simulink library "cpg_lib"  (R2016b)
settings: Solver=VariableStepAuto  StartTime=0.0  StopTime=10.0  RelTol=1e-3  EnableMultiTasking=on
undefined symbols (not defined in the file or in its folder): AFOFS_DIM, c, c_jointstop, CPG, D1G_HAT, DeltaThRef, eref, FmaxGAS, FmaxGLU, FmaxHAM, FmaxHFL, FmaxSOL, FmaxTA, FmaxVAS, GainDeltaTheta, GainGAS, GainGLU, GainHAM, GainHAMHFL, GainHFL, GainKneOverExt, GainSOL, GainSOLTA, GainTA, GainVAS, GroundFunction, K, K_swing, KneePh23Offset, LceOffsetHAM, LceOffsetHFL, LceOffsetTA, left, LongDelay, loptGAS, loptGLU, loptHAM, loptHFL, loptSOL, loptTA, loptVAS, lslackGAS, lslackGLU, lslackHAM, lslackHFL, lslackSOL, lslackTA, lslackVAS, massGAS, massGLU, massHAM, massHFL, massSOL, massTA, massVAS, MidDelay, N, N_record, N_start, phi12_LowLimit ... (+67)
undefined symbols (not defined in the file): NominalShape1
libraries: cpg_lib x36, simulink_extras x14, simulink x5, nmc x3
(part 1 of 4)
settings Model: Creator=efx  LastModifiedBy=brugtjh
settings DataIOCC: LimitDataPoints=on
settings OptimizationCC: LifeSpan=inf
settings DebuggingCC: AllowSymbolicDim=off  SFUnexpectedBacktrackingDiag=warning  SFNoUnconditionalDefaultTransitionDiag=warning  SFExecutionAtInitializationDiag=none
settings ModelReferenceCC: PropagateSignalLabelsOutOfModel=off
settings GRTTargetCC: TargetLangStandard=C89/C90 (ANSI)
settings ConfigComp: CovMetricSettings=dw  CovHtmlReporting=on  CovSaveCumulativeToWorkspaceVar=on  CovSaveSingleToWorkspaceVar=on  CovExternalEMLEnable=off

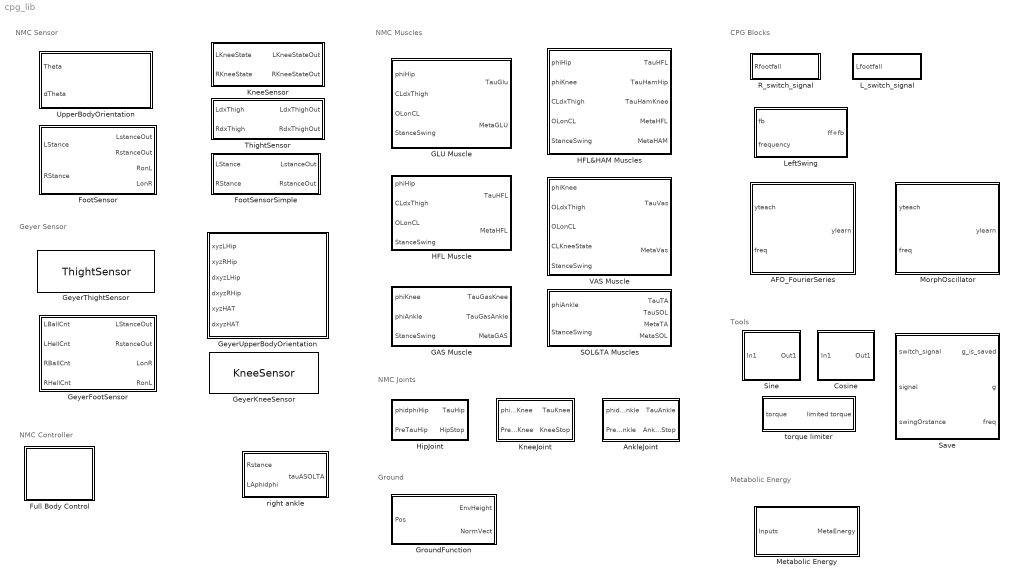
== system cpg_lib ==
  note: NMC Joints
  note: NMC Muscles
  note: Geyer Sensor
  note: NMC Sensor
  note: Tools
  note: CPG Blocks
  note: NMC Controller
  note: Metabolic Energy
  note: Ground
  AFO_FourierSeries : Subsystem
  AnkleJoint : Subsystem
  Cosine : Subsystem
  FootSensor : Subsystem
  FootSensorSimple : Subsystem
  Full Body Control : Subsystem
  GAS Muscle : Subsystem
  GLU Muscle : Subsystem
  GeyerFootSensor : Subsystem
  GeyerKneeSensor : cpg_lib/KneeSensor
  GeyerThightSensor : cpg_lib/ThightSensor
  GeyerUpperBodyOrientation : Subsystem
  GroundFunction : Subsystem
  "HFL Muscle " : Subsystem
  HFL&HAM Muscles : Subsystem
  HipJoint : Subsystem
  KneeJoint : Subsystem
  KneeSensor : Subsystem
  L_switch_signal : Subsystem
  LeftSwing : Subsystem  InitFcn=CPG.initCurrent();  StopFcn=CPG.saveCurrent();  mask{SaveName=NominalShape1}
      mask prompts: SaveName "Signal nominal shape name"
      mask init:
      | evalin('base','CPG.initCPG();');
      settings: CopyFcn=CPG.initCPG_automaticName();
  Metabolic Energy : Subsystem
  MorphOscillator : Subsystem
  R_switch_signal : Subsystem
  SOL&TA Muscles : Subsystem
  Save : Subsystem
  Sine : Subsystem
  ThightSensor : Subsystem
  UpperBodyOrientation : Subsystem
  VAS Muscle : Subsystem
  right ankle : Subsystem
  torque limiter : Subsystem

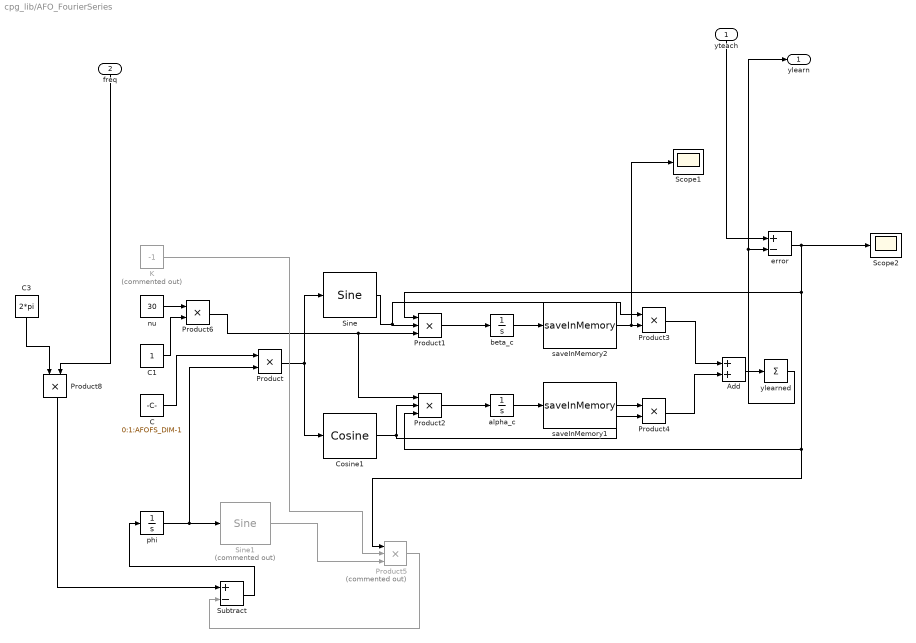
== system cpg_lib/AFO_FourierSeries ==
  yteach : Inport
  freq : Inport  Port=2
  Add : Sum
  C : Constant  Value=0:1:AFOFS_DIM-1
  C1 : Constant
  C3 : Constant  Value=2*pi
  Cosine1 : cpg_lib/Cosine
  K : Constant  Commented=on  Value=-1
  Product{,3..4,6,8} (5 alike) : Product
  Product1 : Product  Inputs=3
  Product2 : Product  Inputs=3
  Product5 : Product  Commented=on  Inputs=3
  Scope1 : Scope
  Scope2 : Scope
  Sine : cpg_lib/Sine
  Sine1 : simulink/Lookup Tables/Sine  Commented=on  Formula=sin(2*pi*u)  NumDataPoints=(2^5)+1  OutputWordLength=16  InternalRulePriority=Speed
  Subtract : Sum  Inputs=+-
  alpha_c : Integrator
  beta_c : Integrator
  error : Sum  Inputs=+-
  nu : Constant  Value=30
  phi : Integrator
  saveInMemory1 : cpg_lib/saveInMemory
  saveInMemory2 : cpg_lib/saveInMemory
  ylearned : Sum  Inputs=+
  ylearn : Outport
  wires:
  saveInMemory2/1 -> Product3/2, Scope1/1
  saveInMemory1/1 -> Product4/1
  yteach/1 -> error/1
  Subtract/1 -> phi/1
  Product6/1 -> Product2/1, Product1/3
  Sine1/1 -> Product5/3
  nu/1 -> Product6/1
  C1/1 -> Product6/2
  Product/1 -> Cosine1/1, Sine/1
  Product1/1 -> beta_c/1
  Product2/1 -> alpha_c/1
  beta_c/1 -> saveInMemory2/1
  alpha_c/1 -> saveInMemory1/1
  Product3/1 -> Add/1
  Product4/1 -> Add/2
  Add/1 -> ylearned/1
  ylearned/1 -> ylearn/1, error/2
  K/1 -> Product5/2
  error/1 -> Product1/1, Product2/3, Product5/1, Scope2/1
  Product5/1 -> Subtract/2
  Product8/1 -> Subtract/1
  phi/1 -> Sine1/1, Product/2
  C/1 -> Product/1
  Sine/1 -> Product1/2, Product3/1
  Cosine1/1 -> Product2/2, Product4/2
  freq/1 -> Product8/2
  C3/1 -> Product8/1

== system cpg_lib/AnkleJoint ==
  note: Ankle Joint
  phidphiAnkle : Inport
  PreTauAnkle : Inport  Port=2
  " Ankle Joint Limits" : Subsystem
  Demux : Demux  Outputs=2
  GotoDisabler_Component1 : nmc/GotoDisabler_Component  GotoTag=DisableNMC_JointLimits
  Sum : Sum  Inputs=|++
  Sum of Elements : Sum  Inputs=+
  TauAnkle : Outport
  AnkleStop : Outport  Port=2
  wires:
  Demux/1 -> " Ankle Joint Limits"/1(phi [rad])
  Demux/2 -> " Ankle Joint Limits"/2(dphi [rad/s])
  PreTauAnkle/1 -> Sum of Elements/1
  phidphiAnkle/1 -> Demux/1
  Sum/1 -> TauAnkle/1
  Sum of Elements/1 -> Sum/2
  " Ankle Joint Limits"/1(M_stop [Nm]) -> GotoDisabler_Component1/1
  GotoDisabler_Component1/1 -> Sum/1, AnkleStop/1

== system cpg_lib/Cosine ==
  In1 : Inport
  MATLAB Function1 : MATLAB Function  TreatAsAtomicUnit=on
  Out1 : Outport
  wires:
  In1/1 -> MATLAB Function1/1(t)
  MATLAB Function1/1(y) -> Out1/1

== system cpg_lib/FootSensor ==
  note: Body Mechanics Layer Interface
      | (Foot Skin Sensors)
  LStance : Inport
  RStance : Inport  Port=2
  Data Type1 : DataTypeConversion  OutDataTypeStr=double
  Data Type3 : DataTypeConversion  OutDataTypeStr=double
  L Stance afferent delay : TransportDelay  DelayTime=MidDelay
  R Stance afferent delay : TransportDelay  DelayTime=MidDelay
  Terminator : Terminator
  cross_infulence : Subsystem
  LstanceOut : Outport
  RstanceOut : Outport  Port=2
  RonL : Outport  Port=3
  LonR : Outport  Port=4
  wires:
  cross_infulence/3(LonR) -> LonR/1
  L Stance afferent delay/1 -> cross_infulence/1(LStance), LstanceOut/1
  R Stance afferent delay/1 -> cross_infulence/2(RStance), RstanceOut/1
  cross_infulence/2(Flight) -> Terminator/1
  cross_infulence/1(RonL) -> RonL/1
  RStance/1 -> Data Type3/1
  LStance/1 -> Data Type1/1
  Data Type3/1 -> R Stance afferent delay/1
  Data Type1/1 -> L Stance afferent delay/1

== system cpg_lib/FootSensorSimple ==
  note: Body Mechanics Layer Interface
      | (Foot Skin Sensors)
  LStance : Inport
  RStance : Inport  Port=2
  L Stance afferent delay : TransportDelay  DelayTime=MidDelay
  R Stance afferent delay : TransportDelay  DelayTime=MidDelay
  LstanceOut : Outport
  RstanceOut : Outport  Port=2
  wires:
  LStance/1 -> L Stance afferent delay/1
  RStance/1 -> R Stance afferent delay/1
  L Stance afferent delay/1 -> LstanceOut/1
  R Stance afferent delay/1 -> RstanceOut/1

== system cpg_lib/Full Body Control ==
  Left Side : Subsystem
  Right Side : Subsystem
  Sensors : Subsystem

== system cpg_lib/GAS Muscle ==
  note: GAS Muscle
  phiKnee : Inport
  phiAnkle : Inport  Port=2
  StanceSwing : Inport  Port=3
  "GAS Actuation " : Subsystem
  GAS Control : Subsystem
  TauGasKnee : Outport
  TauGasAnkle : Outport  Port=2
  MetaGAS : Outport  Port=3
  wires:
  phiAnkle/1 -> "GAS Actuation "/2(phiAnkle)
  "GAS Actuation "/1(TauGasKnee) -> TauGasKnee/1
  "GAS Actuation "/2(TauGasAnkle) -> TauGasAnkle/1
  "GAS Actuation "/3(FmGas) -> GAS Control/1(FmGAS)
  StanceSwing/1 -> GAS Control/2(StanceSwing)
  phiKnee/1 -> "GAS Actuation "/1(phiKnee)
  GAS Control/1(StimGAS) -> "GAS Actuation "/3(StimGas)
  "GAS Actuation "/4(MetaEnergy) -> MetaGAS/1

== system cpg_lib/GLU Muscle ==
  note: GLU Muscle
  phiHip : Inport
  CLdxThigh : Inport  Port=2
  OLonCL : Inport  Port=3
  StanceSwing : Inport  Port=4
  GLU Actuation : Subsystem
  GLU Control : Subsystem
  TauGlu : Outport
  MetaGLU : Outport  Port=2
  wires:
  GLU Actuation/2(FmGlu) -> GLU Control/1(FmGlu)
  OLonCL/1 -> GLU Control/5(OLonCL)
  GLU Control/1(StimGlu) -> GLU Actuation/2(StimGlu)
  [ThetaDelayed] -> GLU Control/2(Theta)
  [dThetaDelayed] -> GLU Control/3(dTheta)
  phiHip/1 -> GLU Actuation/1(phiHip)
  CLdxThigh/1 -> GLU Control/4(CLdxThigh)
  StanceSwing/1 -> GLU Control/6(StanceSwing)
  GLU Actuation/1(TauGlu) -> TauGlu/1
  GLU Actuation/3(MetaEnergy) -> MetaGLU/1

== system cpg_lib/GeyerFootSensor ==
  note: Muscle
      | Actuation
      | Layer
      | Interface
      | (Right
      | Muscle
      | Sensors)
  note: Muscle
      | Actuation
      | Layer
      | Interface
      | (Left
      | Muscle
      | Sensors)
  note: Body Mechanics Layer Interface
      | (Foot Skin Sensors)
  LBallCnt : Inport
  LHellCnt : Inport  Port=2
  RBallCnt : Inport  Port=3
  RHellCnt : Inport  Port=4
  Cross Influence Detection : Subsystem
  L Stance afferent delay : TransportDelay  DelayTime=MidDelay
  Left Stance? : Logic  Operator=OR  AllPortsSameDT=off
  R Stance afferent delay : TransportDelay  DelayTime=MidDelay
  Right Stance? : Logic  Operator=OR  AllPortsSameDT=off
  Terminator : Terminator
  LStanceOut : Outport
  RstanceOut : Outport  Port=2
  LonR : Outport  Port=3
  RonL : Outport  Port=4
  tag scope: LStance=global, RStance=global
  wires:
  Right Stance?/1 -> [RStance], R Stance afferent delay/1
  Left Stance?/1 -> L Stance afferent delay/1, [LStance]
  RBallCnt/1 -> Right Stance?/1
  L Stance afferent delay/1 -> Cross Influence Detection/1(LStance), LStanceOut/1
  Cross Influence Detection/2(Flight) -> Terminator/1
  Cross Influence Detection/1(RonL) -> RonL/1
  R Stance afferent delay/1 -> Cross Influence Detection/2(RStance), RstanceOut/1
  Cross Influence Detection/3(LonR) -> LonR/1
  RHellCnt/1 -> Right Stance?/2
  LBallCnt/1 -> Left Stance?/1
  LHellCnt/1 -> Left Stance?/2

== system cpg_lib/GeyerUpperBodyOrientation ==
  note: Upper Body Orientation
  xyzLHip : Inport
  xyzRHip : Inport  Port=2
  dxyzLHip : Inport  Port=3
  dxyzRHip : Inport  Port=4
  xyzHAT : Inport  Port=5
  dxyzHAT : Inport  Port=6
  " Mean Hip Speed" : Gain  Gain=1/2
  Body Pitch loop delay : TransportDelay  DelayTime=ShortDelay
  Body Pitch loop delay. : TransportDelay  DelayTime=ShortDelay
  "Dx, Dy" : Selector  InputPortWidth=3  IndexOptions=Index vector (dialog)  Indices=[1 2]  OutputSizes=1
  Mean Hip Position : Gain  Gain=1/2
  Mux2 : Mux  Inputs=2
  Sum1 : Sum
  Sum2 : Sum
  Sum4 : Sum  Inputs=-+
  Sum5 : Sum  Inputs=+-
  Theta : Fcn  Expr=atan2(u(1),u(2))
  dDx : Selector  InputPortWidth=3  IndexOptions=Index vector (dialog)  Indices=[1 2]  OutputSizes=1
  dTheta : Fcn  Expr=( u(2)*u(3) - u(1)*u(4) ) / D1G_HAT^2
  tag scope: ThetaDelayed=global, dThetaDelayed=global, theta=global
  wires:
  Sum4/1 -> "Dx, Dy"/1
  dxyzHAT/1 -> Sum5/1
  Sum5/1 -> dDx/1
  dDx/1 -> Mux2/2
  Mux2/1 -> dTheta/1
  xyzLHip/1 -> Sum1/1
  Sum1/1 -> Mean Hip Position/1
  Sum2/1 -> " Mean Hip Speed"/1
  Mean Hip Position/1 -> Sum4/1
  " Mean Hip Speed"/1 -> Sum5/2
  Theta/1 -> [theta], Body Pitch loop delay/1
  dTheta/1 -> Body Pitch loop delay./1
  "Dx, Dy"/1 -> Mux2/1, Theta/1
  xyzRHip/1 -> Sum1/2
  dxyzLHip/1 -> Sum2/1
  xyzHAT/1 -> Sum4/2
  dxyzRHip/1 -> Sum2/2
  Body Pitch loop delay/1 -> [ThetaDelayed]
  Body Pitch loop delay./1 -> [dThetaDelayed]

== system cpg_lib/GroundFunction ==
  Pos : Inport
  GroundFunction : Constant  Value=GroundFunction
  HeightFunction : Fcn  Expr=(a1*u(1)+c2) * (u(1)>=b2) + ((a1/(2*(b2-b1)))*(u(1)*u(1))-((a1*b1)/(b2-b1))*u(1)+c1) *(u(1)>=b1) * (u(1)<b2)
  Multiport Switch : MultiPortSwitch  Inputs=2
  Multiport Switch1 : MultiPortSwitch  Inputs=2
  Mux : Mux  Inputs=2
  NormalFunction : Fcn  Expr=0 * u(1)
  RotFunction : Fcn  Expr=cos(theta)*u(1) - sin(theta)*u(3)
  Zero_Ground : Constant  Value=0
  nVec1 : Constant  Value=[0 1 0]
  nVec2 : Constant  Value=[1 0]
  EnvHeight : Outport
  NormVect : Outport  Port=2
  wires:
  RotFunction/1 -> NormalFunction/1, HeightFunction/1
  Pos/1 -> RotFunction/1
  Mux/1 -> Multiport Switch1/2
  nVec2/1 -> Mux/2
  NormalFunction/1 -> Mux/1
  Multiport Switch/1 -> EnvHeight/1  "EnvHeight"
  Multiport Switch1/1 -> NormVect/1
  Zero_Ground/1 -> Multiport Switch/3
  HeightFunction/1 -> Multiport Switch/2
  nVec1/1 -> Multiport Switch1/3
  GroundFunction/1 -> Multiport Switch/1, Multiport Switch1/1

== system cpg_lib/HFL Muscle  ==
  note: HFL Muscle
  phiHip : Inport
  CLdxThigh : Inport  Port=2
  OLonCL : Inport  Port=3
  StanceSwing : Inport  Port=4
  HFL Actuation : Subsystem
  HFL Control : Subsystem
  TauHFL : Outport
  MetaHFL : Outport  Port=2
  wires:
  HFL Actuation/2(LceHFL) -> HFL Control/1(LceHFL)
  HFL Control/1(StimHFL) -> HFL Actuation/2(StimHFL)
  [ThetaDelayed] -> HFL Control/2(Theta)
  [dThetaDelayed] -> HFL Control/3(dTheta)
  CLdxThigh/1 -> HFL Control/4(CLdxThigh)
  OLonCL/1 -> HFL Control/5(OLonCL)
  StanceSwing/1 -> HFL Control/6(StanceSwing)
  phiHip/1 -> HFL Actuation/1(phiHip)
  HFL Actuation/1(TauHFL) -> TauHFL/1
  HFL Actuation/3(MetaEnergy) -> MetaHFL/1

== system cpg_lib/HFL&HAM Muscles ==
  note: HFL&HAM Muscles
  phiHip : Inport
  phiKnee : Inport  Port=2
  CLdxThigh : Inport  Port=3
  OLonCL : Inport  Port=4
  StanceSwing : Inport  Port=5
  "HAM Actuation " : Subsystem
  HFL Actuation : Subsystem
  HFL&HAM Control : Subsystem
  TauHFL : Outport
  TauHamHip : Outport  Port=2
  TauHamKnee : Outport  Port=3
  MetaHFL : Outport  Port=4
  MetaHAM : Outport  Port=5
  wires:
  HFL&HAM Control/2(StimHAM) -> "HAM Actuation "/3(StimHam)
  StanceSwing/1 -> HFL&HAM Control/8(StanceSwing)
  [dThetaDelayed] -> HFL&HAM Control/5(dTheta)
  [ThetaDelayed] -> HFL&HAM Control/4(Theta)
  phiKnee/1 -> "HAM Actuation "/2(phiKnee)
  HFL Actuation/1(TauHFL) -> TauHFL/1
  CLdxThigh/1 -> HFL&HAM Control/6(CLdxThigh)
  "HAM Actuation "/2(TauHamKnee) -> TauHamKnee/1
  phiHip/1 -> "HAM Actuation "/1(phiHip), HFL Actuation/1(phiHip)
  "HAM Actuation "/1(TauHamHip) -> TauHamHip/1
  OLonCL/1 -> HFL&HAM Control/7(OLonCL)
  HFL Actuation/2(LceHFL) -> HFL&HAM Control/1(LceHFL)
  "HAM Actuation "/4(FmHam) -> HFL&HAM Control/3(FmHam)
  "HAM Actuation "/3(LceHam) -> HFL&HAM Control/2(LceHam)
  HFL&HAM Control/1(StimHFL) -> HFL Actuation/2(StimHFL)
  HFL Actuation/3(MetaEnergy) -> MetaHFL/1
  "HAM Actuation "/5(MetaEnergy) -> MetaHAM/1

== system cpg_lib/HipJoint ==
  note: Hip Joint
  phidphiHip : Inport
  PreTauHip : Inport  Port=2
  Demux2 : Demux  Outputs=2
  GotoDisabler_Component1 : nmc/GotoDisabler_Component  GotoTag=DisableNMC_JointLimits
  Hip Joint Limits : Subsystem
  Sum of Elements : Sum  Inputs=+
  Sum16 : Sum  Inputs=|++
  TauHip : Outport
  HipStop : Outport  Port=2
  wires:
  phidphiHip/1 -> Demux2/1
  Demux2/1 -> Hip Joint Limits/1(phi [rad])
  Demux2/2 -> Hip Joint Limits/2(dphi [rad/s])
  Hip Joint Limits/1(M_stop [Nm]) -> GotoDisabler_Component1/1
  Sum16/1 -> TauHip/1
  PreTauHip/1 -> Sum of Elements/1
  Sum of Elements/1 -> Sum16/2
  GotoDisabler_Component1/1 -> HipStop/1, Sum16/1

== system cpg_lib/KneeJoint ==
  note: Knee Joint
  phidphiKnee : Inport
  PreTauKnee : Inport  Port=2
  Demux1 : Demux  Outputs=2
  Gain : Gain  Gain=-1
  GotoDisabler_Component1 : nmc/GotoDisabler_Component  GotoTag=DisableNMC_JointLimits
  Knee Joint Limits : Subsystem
  Sum : Sum  Inputs=|++
  Sum of Elements : Sum  Inputs=+
  TauKnee : Outport
  KneeStop : Outport  Port=2
  wires:
  Demux1/1 -> Knee Joint Limits/1(phi [rad])
  Demux1/2 -> Knee Joint Limits/2(dphi [rad/s])
  phidphiKnee/1 -> Demux1/1
  Knee Joint Limits/1(M_stop [Nm]) -> GotoDisabler_Component1/1
  PreTauKnee/1 -> Sum of Elements/1
  Sum of Elements/1 -> Gain/1
  Gain/1 -> Sum/2
  Sum/1 -> TauKnee/1
  GotoDisabler_Component1/1 -> KneeStop/1, Sum/1

== system cpg_lib/KneeSensor ==
  note: Body Mechanics Layer Interface
      | (Knee Sensors)
  LKneeState : Inport
  RKneeState : Inport  Port=2
  Demux1 : Demux  Outputs=2
  Demux2 : Demux  Outputs=2
  L Knee loop delay : TransportDelay  DelayTime=MidDelay
  Mux1 : Mux  Inputs=2
  Mux6 : Mux  Inputs=2
  R Knee loop delay : TransportDelay  DelayTime=MidDelay
  Stimulation Bias1 : Constant  Value=KneePh23Offset
  Stimulation Bias10 : Constant  Value=KneePh23Offset
  Sum1 : Sum  Inputs=-+|  SaturateOnIntegerOverflow=on  InputSameDT=on  OutDataTypeStr=Inherit: Same as first input
  Sum6 : Sum  Inputs=-+|  SaturateOnIntegerOverflow=on  InputSameDT=on  OutDataTypeStr=Inherit: Same as first input
  map (-pi,pi] to [0,2pi)1 : Fcn  Expr=u(1)*(u(1)>0)*(u(2)>0)
  map (-pi,pi] to [0,2pi)2 : Fcn  Expr=u(1)*(u(1)>0)*(u(2)>0)
  LKneeStateOut : Outport
  RKneeStateOut : Outport  Port=2
  wires:
  RKneeState/1 -> Demux2/1
  Demux2/1 -> Sum6/2
  Demux2/2 -> Mux6/2
  Sum6/1 -> Mux6/1
  Mux6/1 -> map (-pi,pi] to [0,2pi)1/1
  map (-pi,pi] to [0,2pi)1/1 -> R Knee loop delay/1
  Stimulation Bias10/1 -> Sum6/1
  R Knee loop delay/1 -> RKneeStateOut/1
  LKneeState/1 -> Demux1/1
  Demux1/1 -> Sum1/2
  Demux1/2 -> Mux1/2
  Sum1/1 -> Mux1/1
  Mux1/1 -> map (-pi,pi] to [0,2pi)2/1
  map (-pi,pi] to [0,2pi)2/1 -> L Knee loop delay/1
  Stimulation Bias1/1 -> Sum1/1
  L Knee loop delay/1 -> LKneeStateOut/1

== system cpg_lib/L_switch_signal ==
  Lfootfall : Inport
  Memory : Memory
  Subtract : Sum  Inputs=+-
  tag scope: CPG_leftSwitchSignal=global
  wires:
  Lfootfall/1 -> Memory/1, Subtract/1
  Memory/1 -> Subtract/2
  Subtract/1 -> [CPG_leftSwitchSignal]

== system cpg_lib/LeftSwing ==
  fb : Inport
  frequency : Inport  Port=2
  AlreadySavedInWorkspace : Constant  Value=CPG.Signals.NominalShape1.Enabled
  CPG : Subsystem
  ChooseOutput : Switch  Criteria=u2 > Threshold  Threshold=0.5
  GenerateAndSaveNominalShape : Subsystem
  LeftOrRight : Subsystem
  Logical Operator : Logic  Operator=NOT  Inputs=1  AllPortsSameDT=off  OutDataTypeStr=boolean
  leftOrright : Constant  Value=left
  swingOrstance : Constant  Value=swing
  ff+fb : Outport
  wires:
  LeftOrRight/1(switch_signal) -> GenerateAndSaveNominalShape/1(switch_signal)
  leftOrright/1 -> LeftOrRight/1(side)
  ChooseOutput/1 -> ff+fb/1
  frequency/1 -> CPG/1(freq)
  CPG/1(y) -> ChooseOutput/1
  Logical Operator/1 -> GenerateAndSaveNominalShape/Enable
  swingOrstance/1 -> GenerateAndSaveNominalShape/3(swingOrstance)
  fb/1 -> ChooseOutput/3, GenerateAndSaveNominalShape/2(signal)
  AlreadySavedInWorkspace/1 -> CPG/Enable, ChooseOutput/2, Logical Operator/1

== system cpg_lib/Metabolic Energy ==
  Inputs : Inport
  Demux : Demux  Outputs=10
  Lse : Terminator
  Metabolic Energy : MATLAB Function  TreatAsAtomicUnit=on
  MetaEnergy : Outport
  wires:
  Inputs/1 -> Demux/1
  Metabolic Energy/1(E) -> MetaEnergy/1
  Demux/4 -> Lse/1
  Demux/1 -> Metabolic Energy/1(Fmtc)
  Demux/2 -> Metabolic Energy/2(Lce)
  Demux/3 -> Metabolic Energy/3(Vce)
  Demux/5 -> Metabolic Energy/4(A)
  Demux/6 -> Metabolic Energy/5(Fact)
  Demux/7 -> Metabolic Energy/6(stim)
  Demux/8 -> Metabolic Energy/7(Lopt)
  Demux/9 -> Metabolic Energy/8(mass)
  Demux/10 -> Metabolic Energy/9(typeI_fiber)

== system cpg_lib/MorphOscillator ==
  yteach : Inport
  freq : Inport  Port=2
  Digital Clock : DigitalClock  SampleTime=0.001
  MATLAB Function : MATLAB Function  TreatAsAtomicUnit=on
  ylearn : Outport  SampleTime=0.001
  wires:
  freq/1 -> MATLAB Function/2(freq)
  yteach/1 -> MATLAB Function/1(g)
  Digital Clock/1 -> MATLAB Function/3(t)
  MATLAB Function/1(y) -> ylearn/1

== system cpg_lib/R_switch_signal ==
  Rfootfall : Inport
  Memory : Memory
  Subtract : Sum  Inputs=+-
  tag scope: CPG_rightSwitchSignal=global
  wires:
  Rfootfall/1 -> Subtract/1, Memory/1
  Memory/1 -> Subtract/2
  Subtract/1 -> [CPG_rightSwitchSignal]

== system cpg_lib/SOL&TA Muscles ==
  note: SOL&TA Muscles
  phiAnkle : Inport
  StanceSwing : Inport  Port=2
  SOL Actuation : Subsystem
  SOL&TA Control : Subsystem
  TA Actuation : Subsystem
  TauTA : Outport
  TauSOL : Outport  Port=2
  MetaTA : Outport  Port=3
  MetaSOL : Outport  Port=4
  wires:
  TA Actuation/2(TauTa) -> TauTA/1
  phiAnkle/1 -> SOL Actuation/1(phiAnkle), TA Actuation/1(phiAnkle)
  TA Actuation/1(LceTA) -> SOL&TA Control/1(LceTA)
  StanceSwing/1 -> SOL&TA Control/3(StanceSwing)
  SOL&TA Control/1(StimTA) -> TA Actuation/2(StimTA)
  SOL&TA Control/2(StimSOL) -> SOL Actuation/2(StimSOL)
  SOL Actuation/1(TauSOL) -> TauSOL/1
  SOL Actuation/2(FmSOL) -> SOL&TA Control/2(FmSOL)
  TA Actuation/3(MetaEnergy) -> MetaTA/1
  SOL Actuation/3(MetaEnergy) -> MetaSOL/1

== system cpg_lib/Save ==
  switch_signal : Inport
  signal : Inport  Port=2
  "swingOrstance " : Inport  Port=3
  N_record : Constant  Value=N_record
  N_start : Constant  Value=N_start
  save : Stateflow chart  TreatAsAtomicUnit=on
  g_is_saved : Outport
  g : Outport  Port=2
  freq : Outport  Port=3
  wires:
  save/3(saved) -> g_is_saved/1
  "swingOrstance "/1 -> save/5(swingOrstance)
  save/1(g) -> g/1
  N_start/1 -> save/2(N_start)
  save/2(freq) -> freq/1
  signal/1 -> save/4(signal)
  N_record/1 -> save/3(N_record)
  switch_signal/1 -> save/1(switch_signal)

== system cpg_lib/Sine ==
  In1 : Inport
  MATLAB Function1 : MATLAB Function  TreatAsAtomicUnit=on
  Out1 : Outport
  wires:
  MATLAB Function1/1(y) -> Out1/1
  In1/1 -> MATLAB Function1/1(t)

== system cpg_lib/ThightSensor ==
  note: Body Mechanics Layer Interface
      | (Thigh Body Load Sensors)
  LdxThigh : Inport
  RdxThigh : Inport  Port=2
  L Thigh afferent delay : TransportDelay  DelayTime=ShortDelay
  R Thigh afferent delay : TransportDelay  DelayTime=ShortDelay
  smooth : TransferFcn  Denominator=[0.02 1]
  smooth1 : TransferFcn  Denominator=[0.02 1]
  LdxThighOut : Outport
  RdxThighOut : Outport  Port=2
  wires:
  R Thigh afferent delay/1 -> RdxThighOut/1
  smooth1/1 -> R Thigh afferent delay/1
  LdxThigh/1 -> smooth/1
  smooth/1 -> L Thigh afferent delay/1
  L Thigh afferent delay/1 -> LdxThighOut/1
  RdxThigh/1 -> smooth1/1

== system cpg_lib/UpperBodyOrientation ==
  note: Upper Body Orientation
  Theta : Inport
  dTheta : Inport  Port=2
  Body Pitch loop delay : TransportDelay  DelayTime=ShortDelay
  Body Pitch loop delay. : TransportDelay  DelayTime=ShortDelay
  tag scope: ThetaDelayed=global, dThetaDelayed=global
  wires:
  Theta/1 -> Body Pitch loop delay/1
  dTheta/1 -> Body Pitch loop delay./1
  Body Pitch loop delay/1 -> [ThetaDelayed]
  Body Pitch loop delay./1 -> [dThetaDelayed]

== system cpg_lib/VAS Muscle ==
  note: VAS Muscle
  phiKnee : Inport
  OLdxThigh : Inport  Port=2
  OLonCL : Inport  Port=3
  CLKneeState : Inport  Port=4
  StanceSwing : Inport  Port=5
  "VAS Actuation " : Subsystem
  VAS Control : Subsystem
  TauVas : Outport
  MetaVas : Outport  Port=2
  wires:
  VAS Control/1(StimVAS) -> "VAS Actuation "/2(StimVas)
  "VAS Actuation "/2(FmVas) -> VAS Control/1(FmVAS)
  "VAS Actuation "/1(TauVas) -> TauVas/1
  OLonCL/1 -> VAS Control/3(OLonCL)
  StanceSwing/1 -> VAS Control/5(StanceSwing)
  OLdxThigh/1 -> VAS Control/2(OLdxThigh)
  phiKnee/1 -> "VAS Actuation "/1(phiKnee)
  CLKneeState/1 -> VAS Control/4(CLKneeState)
  "VAS Actuation "/3(MetaEnergy) -> MetaVas/1

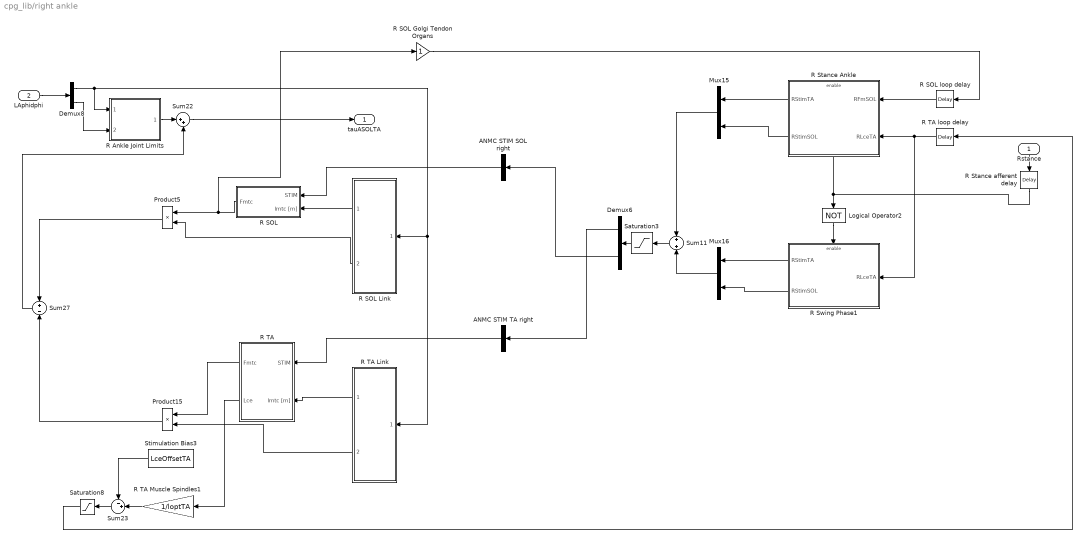
== system cpg_lib/right ankle ==
  Rstance : Inport
  LAphidphi : Inport  Port=2
  ANMC STIM SOL right : Concatenate  NumInputs=1
  ANMC STIM TA right : Concatenate  NumInputs=1
  Demux6 : Demux  Outputs=2
  Demux8 : Demux  Outputs=2
  Logical Operator2 : Logic  Operator=NOT  AllPortsSameDT=off  OutDataTypeStr=boolean
  Mux15 : Mux  Inputs=2
  Mux16 : Mux  Inputs=2
  Product15 : Product  RndMeth=Zero
  Product5 : Product  RndMeth=Zero
  R Ankle Joint Limits : Subsystem
  R SOL : Subsystem
  R SOL Golgi Tendon Organs : Gain
  R SOL Link : Subsystem
  R SOL loop delay : TransportDelay  DelayTime=LongDelay
  R Stance afferent delay : TransportDelay  DelayTime=MidDelay
  R Stance Ankle : Subsystem  TreatAsAtomicUnit=on
  R Swing Phase1 : Subsystem  TreatAsAtomicUnit=on
  R TA : Subsystem
  R TA Muscle Spindles1 : Gain  Gain=1/loptTA
  R TA Link : Subsystem
  R TA loop delay : TransportDelay  DelayTime=LongDelay
  Saturation3 : Saturate  UpperLimit=1  LowerLimit=0.01  ZeroCross=off
  Saturation8 : Saturate  UpperLimit=inf  LowerLimit=0  ZeroCross=off
  Stimulation Bias3 : Constant  Value=LceOffsetTA
  Sum11 : Sum
  Sum22 : Sum  Inputs=|++
  Sum23 : Sum  Inputs=-+|  SaturateOnIntegerOverflow=on  InputSameDT=on  OutDataTypeStr=Inherit: Same as first input
  Sum27 : Sum  Inputs=+-
  tauASOLTA : Outport
  wires:
  Product15/1 -> Sum27/2
  R TA/2(Lce) -> R TA Muscle Spindles1/1
  R TA Link/1(lmtc [m]) -> R TA/2(lmtc [m])
  R TA/1(Fmtc) -> Product15/1
  Product5/1 -> Sum27/1
  Demux8/2 -> R Ankle Joint Limits/2(dphi [rad/s])
  Demux8/1 -> R Ankle Joint Limits/1(phi [rad]), R TA Link/1(phi12 [rad]), R SOL Link/1(phi12 [rad])
  LAphidphi/1 -> Demux8/1
  R Ankle Joint Limits/1(M_stop [Nm]) -> Sum22/1
  Sum27/1 -> Sum22/2
  Sum23/1 -> Saturation8/1
  R TA Link/2(lever [m]) -> Product15/2
  R TA Muscle Spindles1/1 -> Sum23/2
  R SOL/1(Fmtc) -> R SOL Golgi Tendon Organs/1, Product5/1
  R SOL Link/2(lever [m]) -> Product5/2
  Sum22/1 -> tauASOLTA/1
  Stimulation Bias3/1 -> Sum23/1
  R SOL Link/1(lmtc [m]) -> R SOL/2(lmtc [m])
  Saturation3/1 -> Demux6/1
  R Swing Phase1/1(RStimTA) -> Mux16/1
  Logical Operator2/1 -> R Swing Phase1/Enable
  Mux16/1 -> Sum11/2
  Saturation8/1 -> R TA loop delay/1
  Sum11/1 -> Saturation3/1
  R SOL loop delay/1 -> R Stance Ankle/1(RFmSOL)
  R SOL Golgi Tendon Organs/1 -> R SOL loop delay/1
  R Stance Ankle/1(RStimTA) -> Mux15/1
  R Stance afferent delay/1 -> R Stance Ankle/Enable, Logical Operator2/1
  Mux15/1 -> Sum11/1
  R Swing Phase1/2(RStimSOL) -> Mux16/2
  R TA loop delay/1 -> R Swing Phase1/1(RLceTA), R Stance Ankle/2(RLceTA)
  R Stance Ankle/2(RStimSOL) -> Mux15/2
  Rstance/1 -> R Stance afferent delay/1
  Demux6/2 -> ANMC STIM SOL right/1
  ANMC STIM SOL right/1 -> R SOL/1(STIM)
  Demux6/1 -> ANMC STIM TA right/1
  ANMC STIM TA right/1 -> R TA/1(STIM)

== system cpg_lib/torque limiter ==
  torque : Inport
  ANMC limtorque right : Concatenate  NumInputs=1
  ANMC torque ratio right : Constant  Value=0
  Gain : Gain  Gain=-1
  Product : Product
  Saturation : Saturate  UpperLimit=1  LowerLimit=0
  limited torque : Outport
  wires:
  Gain/1 -> Product/1
  ANMC torque ratio right/1 -> Saturation/1
  Saturation/1 -> Gain/1
  torque/1 -> Product/2
  Product/1 -> ANMC limtorque right/1
  ANMC limtorque right/1 -> limited torque/1

== system cpg_lib/AnkleJoint/ Ankle Joint Limits ==
  note: Ankle Joint Limits
  phi [rad] : Inport
  dphi [rad/s] : Inport  Port=2
  Gain1 : Gain  Gain=c_jointstop
  Gain2 : Gain  Gain=-1
  Gain3 : Gain  Gain=c_jointstop
  Gain4 : Gain  Gain=1/w_max_jointstop
  Limit Ankle Range : simulink/Logic and Bit Operations/Interval Test  IntervalClosedRight=on  uplimit=phi12_UpLimit + 40*pi/180  IntervalClosedLeft=on  lowlimit=phi12_LowLimit - 40*pi/180  OutDataTypeStr=boolean
  Logical Operator3 : Logic  Operator=NOT  AllPortsSameDT=off  OutDataTypeStr=boolean
  Mux1 : Mux  Inputs=2
  Mux3 : Mux  Inputs=2
  Overextension Torque : Fcn  Expr="- u(1)  *  (1-u(2)) * (u(2)<1) * (u(1)>0)"
  Overflexion Torque : Fcn  Expr="- u(1)  *  (1-u(2)) * (u(2)<1) * (u(1)<0)"
  Stop Simulation1 : Stop
  Sum : Sum  Inputs=|+-
  Sum1 : Sum  Inputs=|+-
  Sum2 : Sum
  overextension angle : Constant  Value=phi12_UpLimit
  overflexion angle : Constant  Value=phi12_LowLimit
  M_stop [Nm] : Outport
  wires:
  Mux3/1 -> Overextension Torque/1
  Gain3/1 -> Mux3/1
  dphi [rad/s]/1 -> Gain4/1
  overextension angle/1 -> Sum/2
  phi [rad]/1 -> Sum/1, Sum1/1, Limit Ankle Range/1
  Sum/1 -> Gain3/1
  Gain4/1 -> Gain2/1, Mux1/2
  Gain1/1 -> Mux1/1
  Sum1/1 -> Gain1/1
  overflexion angle/1 -> Sum1/2
  Mux1/1 -> Overflexion Torque/1
  Sum2/1 -> M_stop [Nm]/1
  Gain2/1 -> Mux3/2
  Overflexion Torque/1 -> Sum2/2
  Overextension Torque/1 -> Sum2/1
  Limit Ankle Range/1 -> Logical Operator3/1
  Logical Operator3/1 -> Stop Simulation1/1

== system cpg_lib/FootSensor/cross_infulence ==
  note: right leg is leading
  note: left leg is leading
  LStance : Inport  OutDataTypeStr=double
  RStance : Inport  Port=2  OutDataTypeStr=double
  DSup ends : HitCross  HitCrossingOffset=0.5  HitCrossingDirection=falling  ZeroCross=off
  Data Type{,1..3} (4 alike) : DataTypeConversion  OutDataTypeStr=double
  Double Support? : Logic  AllPortsSameDT=off
  Double Support?1 : Logic  AllPortsSameDT=off
  Double Support?4 : Logic  AllPortsSameDT=off
  Flight? : Logic  Operator=NOR  AllPortsSameDT=off
  LLeg starts DSup : HitCross  HitCrossingOffset=0.5  HitCrossingDirection=rising  ZeroCross=off
  Memory : Memory
  Memory3 : Memory
  RLeg starts DSup : HitCross  HitCrossingOffset=0.5  HitCrossingDirection=rising  ZeroCross=off
  S-R Flip-Flop : simulink_extras/Flip Flops/S-R Flip-Flop  initial_condition=0
  S-R Flip-Flop1 : simulink_extras/Flip Flops/S-R Flip-Flop  initial_condition=0
  Terminator1 : Terminator
  Terminator2 : Terminator
  RonL : Outport  OutDataTypeStr=double
  Flight : Outport  Port=2  OutDataTypeStr=double
  LonR : Outport  Port=3  OutDataTypeStr=double
  wires:
  Double Support?1/1 -> S-R Flip-Flop1/1
  S-R Flip-Flop/1 -> Data Type1/1
  RLeg starts DSup/1 -> Double Support?1/2
  S-R Flip-Flop/2 -> Terminator1/1
  DSup ends/1 -> S-R Flip-Flop/2, S-R Flip-Flop1/2
  S-R Flip-Flop1/2 -> Terminator2/1
  Memory/1 -> RLeg starts DSup/1
  LStance/1 -> Memory3/1, Double Support?/1, Flight?/1
  LLeg starts DSup/1 -> Double Support?4/1
  Data Type2/1 -> Flight/1
  Double Support?4/1 -> S-R Flip-Flop/1
  Memory3/1 -> LLeg starts DSup/1
  RStance/1 -> Memory/1, Double Support?/2, Flight?/2
  Double Support?/1 -> Data Type/1, Double Support?1/1, Double Support?4/2
  Flight?/1 -> Data Type2/1
  S-R Flip-Flop1/1 -> Data Type3/1
  Data Type/1 -> DSup ends/1
  Data Type1/1 -> LonR/1
  Data Type3/1 -> RonL/1

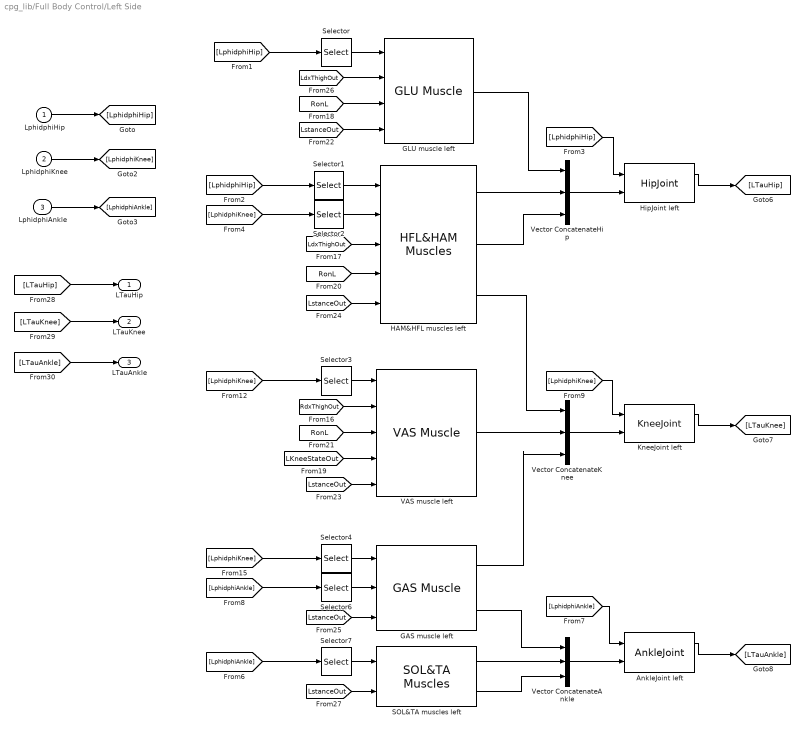
== system cpg_lib/Full Body Control/Left Side ==
  LphidphiHip : Inport
  LphidphiKnee : Inport  Port=2
  LphidphiAnkle : Inport  Port=3
  AnkleJoint left : cpg_lib/AnkleJoint
  GAS muscle left : cpg_lib/GAS Muscle
  GLU muscle left : cpg_lib/GLU Muscle
  HAM&HFL muscles left : cpg_lib/HFL&HAM Muscles
  HipJoint left : cpg_lib/HipJoint
  KneeJoint left : cpg_lib/KneeJoint
  SOL&TA muscles left : cpg_lib/SOL&TA Muscles
  Selector{,1..4,6..7} (7 alike) : Selector  InputPortWidth=2  IndexOptions=Index vector (dialog)  Indices=[1 ]  OutputSizes=1
  VAS muscle left : cpg_lib/VAS Muscle
  Vector ConcatenateAnkle : Concatenate  NumInputs=3
  Vector ConcatenateHip : Concatenate  NumInputs=3
  Vector ConcatenateKnee : Concatenate  NumInputs=3
  LTauHip : Outport
  LTauKnee : Outport  Port=2
  LTauAnkle : Outport  Port=3
  wires:
  [LTauAnkle] -> LTauAnkle/1
  [LTauKnee] -> LTauKnee/1
  [LTauHip] -> LTauHip/1
  LphidphiAnkle/1 -> [LphidphiAnkle]
  LphidphiKnee/1 -> [LphidphiKnee]
  LphidphiHip/1 -> [LphidphiHip]
  [LdxThighOut] -> HAM&HFL muscles left/3
  [RonL] -> GLU muscle left/3
  [LstanceOut] -> GLU muscle left/4
  [LdxThighOut] -> GLU muscle left/2
  AnkleJoint left/1 -> [LTauAnkle]
  KneeJoint left/1 -> [LTauKnee]
  HipJoint left/1 -> [LTauHip]
  [LphidphiKnee] -> Selector2/1
  [LphidphiHip] -> HipJoint left/1
  [LphidphiHip] -> Selector/1
  [LstanceOut] -> VAS muscle left/5
  [LphidphiHip] -> Selector1/1
  [LphidphiAnkle] -> Selector6/1
  Selector2/1 -> HAM&HFL muscles left/2
  HAM&HFL muscles left/2 -> Vector ConcatenateHip/3
  [LstanceOut] -> SOL&TA muscles left/2
  [LphidphiAnkle] -> Selector7/1
  [LstanceOut] -> GAS muscle left/3
  Selector/1 -> GLU muscle left/1
  HAM&HFL muscles left/3 -> Vector ConcatenateKnee/1
  [LKneeStateOut] -> VAS muscle left/4
  [RonL] -> HAM&HFL muscles left/4
  [LphidphiKnee] -> Selector4/1
  [LphidphiKnee] -> Selector3/1
  [RonL] -> VAS muscle left/3
  [LstanceOut] -> HAM&HFL muscles left/5
  GLU muscle left/1 -> Vector ConcatenateHip/1
  HAM&HFL muscles left/1 -> Vector ConcatenateHip/2
  GAS muscle left/1 -> Vector ConcatenateKnee/3
  [LphidphiAnkle] -> AnkleJoint left/1
  VAS muscle left/1 -> Vector ConcatenateKnee/2
  Selector6/1 -> GAS muscle left/2
  Selector3/1 -> VAS muscle left/1
  SOL&TA muscles left/1 -> Vector ConcatenateAnkle/2
  Vector ConcatenateKnee/1 -> KneeJoint left/2
  Vector ConcatenateAnkle/1 -> AnkleJoint left/2
  Selector7/1 -> SOL&TA muscles left/1
  SOL&TA muscles left/2 -> Vector ConcatenateAnkle/3
  [RdxThighOut] -> VAS muscle left/2
  Selector4/1 -> GAS muscle left/1
  Selector1/1 -> HAM&HFL muscles left/1
  [LphidphiKnee] -> KneeJoint left/1
  Vector ConcatenateHip/1 -> HipJoint left/2
  GAS muscle left/2 -> Vector ConcatenateAnkle/1

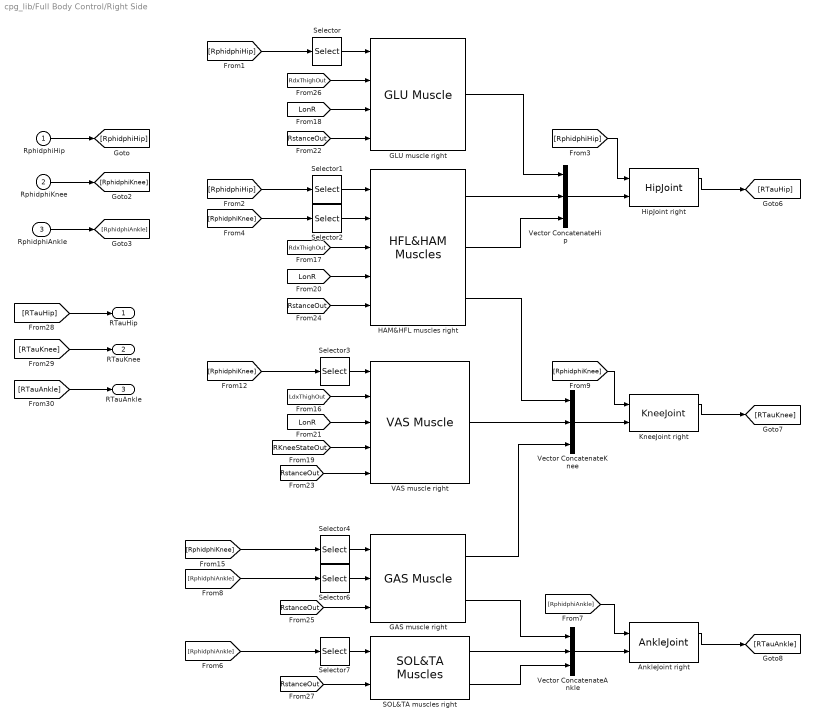
== system cpg_lib/Full Body Control/Right Side ==
  RphidphiHip : Inport
  RphidphiKnee : Inport  Port=2
  RphidphiAnkle : Inport  Port=3
  AnkleJoint right : cpg_lib/AnkleJoint
  GAS muscle right : cpg_lib/GAS Muscle
  GLU muscle right : cpg_lib/GLU Muscle
  HAM&HFL muscles right : cpg_lib/HFL&HAM Muscles
  HipJoint right : cpg_lib/HipJoint
  KneeJoint right : cpg_lib/KneeJoint
  SOL&TA muscles right : cpg_lib/SOL&TA Muscles
  Selector{,1..4,6..7} (7 alike) : Selector  InputPortWidth=2  IndexOptions=Index vector (dialog)  Indices=[1 ]  OutputSizes=1
  VAS muscle right : cpg_lib/VAS Muscle
  Vector ConcatenateAnkle : Concatenate  NumInputs=3
  Vector ConcatenateHip : Concatenate  NumInputs=3
  Vector ConcatenateKnee : Concatenate  NumInputs=3
  RTauHip : Outport
  RTauKnee : Outport  Port=2
  RTauAnkle : Outport  Port=3
  wires:
  [RTauAnkle] -> RTauAnkle/1
  [RTauKnee] -> RTauKnee/1
  [RTauHip] -> RTauHip/1
  RphidphiAnkle/1 -> [RphidphiAnkle]
  RphidphiKnee/1 -> [RphidphiKnee]
  RphidphiHip/1 -> [RphidphiHip]
  [RstanceOut] -> HAM&HFL muscles right/5
  [LonR] -> HAM&HFL muscles right/4
  [RdxThighOut] -> HAM&HFL muscles right/3
  [RstanceOut] -> GLU muscle right/4
  [LonR] -> GLU muscle right/3
  [RdxThighOut] -> GLU muscle right/2
  AnkleJoint right/1 -> [RTauAnkle]
  KneeJoint right/1 -> [RTauKnee]
  HipJoint right/1 -> [RTauHip]
  [RphidphiKnee] -> Selector2/1
  [RphidphiHip] -> HipJoint right/1
  [RphidphiHip] -> Selector/1
  [RstanceOut] -> VAS muscle right/5
  [RphidphiHip] -> Selector1/1
  [RphidphiAnkle] -> Selector6/1
  Selector2/1 -> HAM&HFL muscles right/2
  HAM&HFL muscles right/2 -> Vector ConcatenateHip/3
  [RstanceOut] -> SOL&TA muscles right/2
  [RphidphiAnkle] -> Selector7/1
  [RstanceOut] -> GAS muscle right/3
  Selector/1 -> GLU muscle right/1
  HAM&HFL muscles right/3 -> Vector ConcatenateKnee/1
  [RKneeStateOut] -> VAS muscle right/4
  [RphidphiKnee] -> Selector4/1
  [RphidphiKnee] -> Selector3/1
  [LonR] -> VAS muscle right/3
  GLU muscle right/1 -> Vector ConcatenateHip/1
  HAM&HFL muscles right/1 -> Vector ConcatenateHip/2
  GAS muscle right/1 -> Vector ConcatenateKnee/3
  [RphidphiAnkle] -> AnkleJoint right/1
  VAS muscle right/1 -> Vector ConcatenateKnee/2
  Selector6/1 -> GAS muscle right/2
  Selector3/1 -> VAS muscle right/1
  SOL&TA muscles right/1 -> Vector ConcatenateAnkle/2
  Vector ConcatenateKnee/1 -> KneeJoint right/2
  Vector ConcatenateAnkle/1 -> AnkleJoint right/2
  Selector7/1 -> SOL&TA muscles right/1
  SOL&TA muscles right/2 -> Vector ConcatenateAnkle/3
  [LdxThighOut] -> VAS muscle right/2
  Selector4/1 -> GAS muscle right/1
  Selector1/1 -> HAM&HFL muscles right/1
  [RphidphiKnee] -> KneeJoint right/1
  Vector ConcatenateHip/1 -> HipJoint right/2
  GAS muscle right/2 -> Vector ConcatenateAnkle/1

== system cpg_lib/Full Body Control/Sensors ==
  Theta : Inport
  dTheta : Inport  Port=2
  LdxThigh : Inport  Port=3
  RdxThigh : Inport  Port=4
  LKneeState : Inport  Port=5
  RKneeState : Inport  Port=6
  LStance : Inport  Port=7
  RStance : Inport  Port=8
  FootSensor : cpg_lib/FootSensor
  KneeSensor : cpg_lib/KneeSensor
  ThightSensor : cpg_lib/ThightSensor
  UpperBodyOrientation : cpg_lib/UpperBodyOrientation
  tag scope: LKneeStateOut=global, LdxThighOut=global, LonR=global, LstanceOut=global, RKneeStateOut=global, RdxThighOut=global, RonL=global, RstanceOut=global
  wires:
  RStance/1 -> FootSensor/2
  LStance/1 -> FootSensor/1
  RKneeState/1 -> KneeSensor/2
  LKneeState/1 -> KneeSensor/1
  RdxThigh/1 -> ThightSensor/2
  LdxThigh/1 -> ThightSensor/1
  dTheta/1 -> UpperBodyOrientation/2
  Theta/1 -> UpperBodyOrientation/1
  FootSensor/4 -> [RonL]
  FootSensor/3 -> [LonR]
  FootSensor/2 -> [RstanceOut]
  FootSensor/1 -> [LstanceOut]
  KneeSensor/2 -> [RKneeStateOut]
  KneeSensor/1 -> [LKneeStateOut]
  ThightSensor/1 -> [LdxThighOut]
  ThightSensor/2 -> [RdxThighOut]

== system cpg_lib/GAS Muscle/GAS Actuation  ==
  note: GAS Actuation
  phiKnee : Inport
  phiAnkle : Inport  Port=2
  StimGas : Inport  Port=3
  " GAS" : Subsystem
  " GAS Golgi Tendon Organs" : Gain
  Constant : Constant  Value=loptGAS
  Constant1 : Constant  Value=massGAS
  Constant2 : Constant  Value=t1fGAS
  GAS Link : Subsystem
  GAS loop delay : TransportDelay  DelayTime=LongDelay
  Metabolic Energy : cpg_lib/Metabolic Energy
  Mux : Mux  Inputs=5
  Mux2 : Mux  Inputs=6
  Product2 : Product  RndMeth=Zero
  Product3 : Product  RndMeth=Zero
  TauGasKnee : Outport
  TauGasAnkle : Outport  Port=2
  FmGas : Outport  Port=3
  MetaEnergy : Outport  Port=4
  wires:
  " GAS"/1(Fmtc) -> Product2/1, Product3/1, " GAS Golgi Tendon Organs"/1, Mux2/1
  GAS Link/3(lever12 [m]) -> Product2/2
  GAS Link/2(lever23 [m]) -> Product3/2
  GAS Link/1(lmtu [m]) -> " GAS"/2(lmtc [m])
  Product3/1 -> TauGasKnee/1
  " GAS"/5(A) -> Mux2/5
  " GAS"/4(Lse) -> Mux2/4
  " GAS"/3(Vce) -> Mux2/3
  " GAS"/2(Lce) -> Mux2/2
  phiKnee/1 -> GAS Link/1(phi23 [rad])
  phiAnkle/1 -> GAS Link/2(phi12 [rad])
  Product2/1 -> TauGasAnkle/1
  " GAS Golgi Tendon Organs"/1 -> GAS loop delay/1
  GAS loop delay/1 -> FmGas/1
  " GAS"/6(Fac) -> Mux2/6
  Mux2/1 -> Mux/1
  StimGas/1 -> Mux/2, " GAS"/1(STIM)
  Mux/1 -> Metabolic Energy/1
  Constant2/1 -> Mux/5
  Constant1/1 -> Mux/4
  Constant/1 -> Mux/3
  Metabolic Energy/1 -> MetaEnergy/1

== system cpg_lib/GAS Muscle/GAS Control ==
  note: GAS sControl
  FmGAS : Inport
  StanceSwing : Inport  Port=2
  " Swing Phase" : Subsystem  TreatAsAtomicUnit=on
  "ANMC STIM " : Concatenate  NumInputs=1
  Logical Operator : Logic  Operator=NOT  AllPortsSameDT=off  OutDataTypeStr=boolean
  Saturation17 : Saturate  UpperLimit=1  LowerLimit=0.01  ZeroCross=off
  Stance Phase : Subsystem  TreatAsAtomicUnit=on
  Sum18 : Sum
  StimGAS : Outport
  wires:
  Logical Operator/1 -> " Swing Phase"/Enable
  FmGAS/1 -> Stance Phase/1(FmGAS)
  StanceSwing/1 -> Logical Operator/1, Stance Phase/Enable
  " Swing Phase"/1(StimGAS) -> Sum18/2
  Sum18/1 -> Saturation17/1
  Saturation17/1 -> "ANMC STIM "/1
  Stance Phase/1(StimGAS) -> Sum18/1
  "ANMC STIM "/1 -> StimGAS/1

== system cpg_lib/GLU Muscle/GLU Actuation ==
  note: GLU Actuation
  phiHip : Inport
  StimGlu : Inport  Port=2
  " GLU" : Subsystem
  " GLU Fm loop delay" : TransportDelay  DelayTime=ShortDelay
  Constant : Constant  Value=loptGLU
  Constant1 : Constant  Value=massGLU
  Constant2 : Constant  Value=t1fGLU
  GLU Golgi Tendon Organs : Gain
  GLU Link : Subsystem
  Metabolic Energy : cpg_lib/Metabolic Energy
  Mux : Mux  Inputs=6
  Mux1 : Mux  Inputs=5
  Product6 : Product  RndMeth=Zero
  TauGlu : Outport
  FmGlu : Outport  Port=2
  MetaEnergy : Outport  Port=3
  wires:
  " GLU"/1(Fmtc) -> Mux/1, Product6/1, GLU Golgi Tendon Organs/1
  Product6/1 -> TauGlu/1
  GLU Link/1(lmtu [m]) -> " GLU"/2(lmtc [m])
  GLU Link/2(lever [m]) -> Product6/2
  " GLU"/5(A) -> Mux/5
  GLU Golgi Tendon Organs/1 -> " GLU Fm loop delay"/1
  " GLU"/2(Lce) -> Mux/2
  " GLU"/3(Vce) -> Mux/3
  " GLU"/4(Lse) -> Mux/4
  phiHip/1 -> GLU Link/1(phi34 [rad])
  " GLU Fm loop delay"/1 -> FmGlu/1
  " GLU"/6(Fac) -> Mux/6
  Mux/1 -> Mux1/1
  StimGlu/1 -> Mux1/2, " GLU"/1(STIM)
  Mux1/1 -> Metabolic Energy/1
  Constant2/1 -> Mux1/5
  Constant1/1 -> Mux1/4
  Constant/1 -> Mux1/3
  Metabolic Energy/1 -> MetaEnergy/1

== system cpg_lib/GLU Muscle/GLU Control ==
  note: GLU Control
  FmGlu : Inport
  Theta : Inport  Port=2
  dTheta : Inport  Port=3
  CLdxThigh : Inport  Port=4
  OLonCL : Inport  Port=5
  StanceSwing : Inport  Port=6
  " Swing Phase" : Subsystem  TreatAsAtomicUnit=on
  "ANMC STIM " : Concatenate  NumInputs=1
  Logical Operator : Logic  Operator=NOT  AllPortsSameDT=off  OutDataTypeStr=boolean
  Saturation17 : Saturate  UpperLimit=1  LowerLimit=0.01  ZeroCross=off
  Stance Phase : Subsystem  TreatAsAtomicUnit=on
  Sum18 : Sum
  StimGlu : Outport
  wires:
  Logical Operator/1 -> " Swing Phase"/Enable
  " Swing Phase"/1(StimGLU) -> Sum18/2
  FmGlu/1 -> " Swing Phase"/1(FmGLU)
  Sum18/1 -> Saturation17/1
  Saturation17/1 -> "ANMC STIM "/1
  dTheta/1 -> Stance Phase/2(dTheta [rad/s])
  Theta/1 -> Stance Phase/1(Theta)
  Stance Phase/1(StimGLU) -> Sum18/1
  CLdxThigh/1 -> Stance Phase/3(CLdxThigh [N])
  OLonCL/1 -> Stance Phase/4(OLonCL)
  StanceSwing/1 -> Logical Operator/1, Stance Phase/Enable
  "ANMC STIM "/1 -> StimGlu/1

== system cpg_lib/GeyerFootSensor/Cross Influence Detection ==
  note: left leg is leading
  note: right leg is leading
  note: Double Support Cross Influences
  LStance : Inport  OutDataTypeStr=double
  RStance : Inport  Port=2  OutDataTypeStr=double
  DSup ends : HitCross  HitCrossingOffset=0.5  HitCrossingDirection=falling  ZeroCross=off
  Double Support? : Logic  AllPortsSameDT=off
  Double Support?1 : Logic  AllPortsSameDT=off
  Double Support?4 : Logic  AllPortsSameDT=off
  Flight? : Logic  Operator=NOR  AllPortsSameDT=off
  LLeg starts DSup : HitCross  HitCrossingOffset=0.5  HitCrossingDirection=rising  ZeroCross=off
  Memory : Memory
  Memory3 : Memory
  RLeg starts DSup : HitCross  HitCrossingOffset=0.5  HitCrossingDirection=rising  ZeroCross=off
  S-R Flip-Flop : simulink_extras/Flip Flops/S-R Flip-Flop  initial_condition=0
  S-R Flip-Flop1 : simulink_extras/Flip Flops/S-R Flip-Flop  initial_condition=0
  Terminator1 : Terminator
  Terminator2 : Terminator
  RonL : Outport  OutDataTypeStr=double
  Flight : Outport  Port=2  OutDataTypeStr=double
  LonR : Outport  Port=3  OutDataTypeStr=double
  wires:
  S-R Flip-Flop1/1 -> RonL/1
  Flight?/1 -> Flight/1
  S-R Flip-Flop/1 -> LonR/1
  Double Support?/1 -> DSup ends/1, Double Support?4/2, Double Support?1/1
  RStance/1 -> Flight?/2, Double Support?/2, Memory/1
  Memory3/1 -> LLeg starts DSup/1
  Double Support?4/1 -> S-R Flip-Flop/1
  LLeg starts DSup/1 -> Double Support?4/1
  LStance/1 -> Flight?/1, Double Support?/1, Memory3/1
  Memory/1 -> RLeg starts DSup/1
  S-R Flip-Flop1/2 -> Terminator2/1
  DSup ends/1 -> S-R Flip-Flop1/2, S-R Flip-Flop/2
  S-R Flip-Flop/2 -> Terminator1/1
  RLeg starts DSup/1 -> Double Support?1/2
  Double Support?1/1 -> S-R Flip-Flop1/1

== system cpg_lib/HFL Muscle /HFL Actuation ==
  note: HFL Actuation
  phiHip : Inport
  StimHFL : Inport  Port=2
  " HFL" : Subsystem
  " HFL Muscle Spindles" : Gain  Gain=1/loptHFL
  " HFL Link" : Subsystem
  Constant : Constant  Value=loptHFL
  Constant1 : Constant  Value=massHFL
  Constant2 : Constant  Value=t1fHFL
  Gain : Gain  Gain=-1
  HFL Lce loop delay : TransportDelay  DelayTime=ShortDelay
  Metabolic Energy : cpg_lib/Metabolic Energy
  Mux : Mux  Inputs=5
  Mux10 : Mux  Inputs=6
  Product7 : Product  RndMeth=Zero
  Saturation5 : Saturate  UpperLimit=inf  LowerLimit=0  ZeroCross=off
  Stimulation Bias5 : Constant  Value=LceOffsetHFL
  Sum24 : Sum  Inputs=-+|  SaturateOnIntegerOverflow=on  InputSameDT=on  OutDataTypeStr=Inherit: Same as first input
  TauHFL : Outport
  LceHFL : Outport  Port=2
  MetaEnergy : Outport  Port=3
  wires:
  Stimulation Bias5/1 -> Sum24/1
  " HFL"/1(Fmtc) -> Mux10/1, Product7/2
  " HFL"/2(Lce) -> Mux10/2, " HFL Muscle Spindles"/1
  " HFL Link"/1(lmtu [m]) -> " HFL"/2(lmtc [m])
  " HFL"/5(A) -> Mux10/5
  " HFL Link"/2(lever [m]) -> Product7/1
  " HFL Muscle Spindles"/1 -> Sum24/2
  Sum24/1 -> Saturation5/1
  Saturation5/1 -> HFL Lce loop delay/1
  " HFL"/4(Lse) -> Mux10/4
  " HFL"/3(Vce) -> Mux10/3
  phiHip/1 -> " HFL Link"/1(phi34 [rad])
  Product7/1 -> Gain/1
  Gain/1 -> TauHFL/1
  HFL Lce loop delay/1 -> LceHFL/1
  " HFL"/6(Fac) -> Mux10/6
  Mux10/1 -> Mux/1
  StimHFL/1 -> Mux/2, " HFL"/1(STIM)
  Mux/1 -> Metabolic Energy/1
  Constant2/1 -> Mux/5
  Constant1/1 -> Mux/4
  Constant/1 -> Mux/3
  Metabolic Energy/1 -> MetaEnergy/1

== system cpg_lib/HFL Muscle /HFL Control ==
  note: HFL Control
  LceHFL : Inport
  Theta : Inport  Port=2
  dTheta : Inport  Port=3
  CLdxThigh : Inport  Port=4
  OLonCL : Inport  Port=5
  StanceSwing : Inport  Port=6
  "ANMC STIM " : Concatenate  NumInputs=1
  Logical Operator : Logic  Operator=NOT  AllPortsSameDT=off  OutDataTypeStr=boolean
  Saturation17 : Saturate  UpperLimit=1  LowerLimit=0.01  ZeroCross=off
  Stance Phase : Subsystem  TreatAsAtomicUnit=on
  Sum18 : Sum
  Swing Phase : Subsystem  TreatAsAtomicUnit=on
  StimHFL : Outport
  wires:
  Saturation17/1 -> "ANMC STIM "/1
  OLonCL/1 -> Stance Phase/4(OLonCL)
  Swing Phase/1(StimHFL) -> Sum18/2
  Sum18/1 -> Saturation17/1
  StanceSwing/1 -> Stance Phase/Enable, Logical Operator/1
  LceHFL/1 -> Swing Phase/2(LceHFL)
  Stance Phase/1(StimHFL) -> Sum18/1
  CLdxThigh/1 -> Stance Phase/3(CLdxThigh [N])
  Stance Phase/2(Delta_Theta) -> Swing Phase/1(Delta_Theta)
  dTheta/1 -> Stance Phase/2(dTheta [rad/s])
  Theta/1 -> Stance Phase/1(Theta)
  Logical Operator/1 -> Swing Phase/Enable
  "ANMC STIM "/1 -> StimHFL/1

== system cpg_lib/HFL&HAM Muscles/HAM Actuation  ==
  note: HAM Actuation
  phiHip : Inport
  phiKnee : Inport  Port=2
  StimHam : Inport  Port=3
  " HAM Muscle Spindles" : Gain  Gain=1/loptHAM
  " HAM Fm loop delay" : TransportDelay  DelayTime=ShortDelay
  " HAM Link" : Subsystem
  Constant : Constant  Value=loptHAM
  Constant1 : Constant  Value=massHAM
  Constant2 : Constant  Value=t1fHAM
  HAM : Subsystem
  HAM Golgi Tendon Organs : Gain
  HAM Lce loop delay : TransportDelay  DelayTime=ShortDelay
  Metabolic Energy : cpg_lib/Metabolic Energy
  Mux : Mux  Inputs=5
  Mux1 : Mux  Inputs=6
  Product8 : Product  RndMeth=Zero
  Product9 : Product  RndMeth=Zero
  Saturation7 : Saturate  UpperLimit=inf  LowerLimit=0  ZeroCross=off
  Stimulation Bias7 : Constant  Value=LceOffsetHAM
  Sum26 : Sum  Inputs=-+|  SaturateOnIntegerOverflow=on  InputSameDT=on  OutDataTypeStr=Inherit: Same as first input
  TauHamHip : Outport
  TauHamKnee : Outport  Port=2
  LceHam : Outport  Port=3
  FmHam : Outport  Port=4
  MetaEnergy : Outport  Port=5
  wires:
  phiKnee/1 -> " HAM Link"/2(phi23 [rad])
  HAM/1(Fmtc) -> Product9/1, Product8/1, HAM Golgi Tendon Organs/1, Mux1/1
  HAM/2(Lce) -> " HAM Muscle Spindles"/1, Mux1/2
  " HAM Link"/1(lmtu [m]) -> HAM/2(lmtc [m])
  " HAM Link"/2(lever34 [m]) -> Product8/2
  " HAM Link"/3(lever23 [m]) -> Product9/2
  phiHip/1 -> " HAM Link"/1(phi34 [rad])
  HAM/5(A) -> Mux1/5
  Product8/1 -> TauHamHip/1
  HAM Golgi Tendon Organs/1 -> " HAM Fm loop delay"/1
  " HAM Muscle Spindles"/1 -> Sum26/2
  Sum26/1 -> Saturation7/1
  Mux1/1 -> Mux/1
  HAM/4(Lse) -> Mux1/4
  HAM/3(Vce) -> Mux1/3
  Stimulation Bias7/1 -> Sum26/1
  Product9/1 -> TauHamKnee/1
  StimHam/1 -> Mux/2, HAM/1(STIM)
  Saturation7/1 -> HAM Lce loop delay/1
  HAM Lce loop delay/1 -> LceHam/1
  " HAM Fm loop delay"/1 -> FmHam/1
  HAM/6(Fac) -> Mux1/6
  Mux/1 -> Metabolic Energy/1
  Constant2/1 -> Mux/5
  Constant1/1 -> Mux/4
  Constant/1 -> Mux/3
  Metabolic Energy/1 -> MetaEnergy/1

== system cpg_lib/HFL&HAM Muscles/HFL Actuation ==
  note: HFL Actuation
  phiHip : Inport
  StimHFL : Inport  Port=2
  " HFL" : Subsystem
  " HFL Muscle Spindles" : Gain  Gain=1/loptHFL
  " HFL Link" : Subsystem
  Constant : Constant  Value=loptHFL
  Constant1 : Constant  Value=massHFL
  Constant2 : Constant  Value=t1fHFL
  Gain : Gain  Gain=-1
  HFL Lce loop delay : TransportDelay  DelayTime=ShortDelay
  Metabolic Energy : cpg_lib/Metabolic Energy
  Mux : Mux  Inputs=5
  Mux10 : Mux  Inputs=6
  Product7 : Product  RndMeth=Zero
  Saturation5 : Saturate  UpperLimit=inf  LowerLimit=0  ZeroCross=off
  Stimulation Bias5 : Constant  Value=LceOffsetHFL
  Sum24 : Sum  Inputs=-+|  SaturateOnIntegerOverflow=on  InputSameDT=on  OutDataTypeStr=Inherit: Same as first input
  TauHFL : Outport
  LceHFL : Outport  Port=2
  MetaEnergy : Outport  Port=3
  wires:
  Stimulation Bias5/1 -> Sum24/1
  " HFL"/1(Fmtc) -> Product7/2, Mux10/1
  " HFL"/2(Lce) -> " HFL Muscle Spindles"/1, Mux10/2
  " HFL Link"/1(lmtu [m]) -> " HFL"/2(lmtc [m])
  " HFL"/5(A) -> Mux10/5
  " HFL Link"/2(lever [m]) -> Product7/1
  " HFL Muscle Spindles"/1 -> Sum24/2
  Sum24/1 -> Saturation5/1
  Saturation5/1 -> HFL Lce loop delay/1
  " HFL"/4(Lse) -> Mux10/4
  " HFL"/3(Vce) -> Mux10/3
  phiHip/1 -> " HFL Link"/1(phi34 [rad])
  Product7/1 -> Gain/1
  Gain/1 -> TauHFL/1
  HFL Lce loop delay/1 -> LceHFL/1
  Mux10/1 -> Mux/1
  StimHFL/1 -> Mux/2, " HFL"/1(STIM)
  Mux/1 -> Metabolic Energy/1
  Constant2/1 -> Mux/5
  Constant1/1 -> Mux/4
  Constant/1 -> Mux/3
  Metabolic Energy/1 -> MetaEnergy/1
  " HFL"/6(Fac) -> Mux10/6
